simulink model "wheelSuspension"  (R2025a)
settings: Solver=VariableStepAuto  StartTime=0.0  StopTime=10  RelTol=1e-3
undefined symbols (not defined in the file): cs, ks, mass_payload, mass_robot, robot_height
settings Model: DataDictionary=Constants.sldd  Creator=yaremadzulynsky  LastModifiedBy=yaremadzulynsky

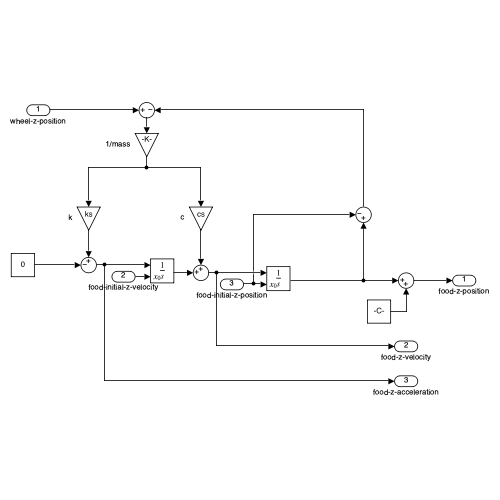
[thumbnail: Simulink's stored preview of the top-level diagram]
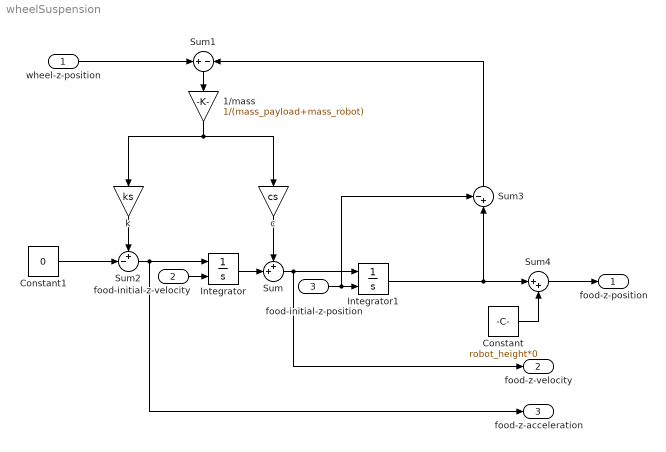
== system wheelSuspension ==
  wheel-z-position : Inport
  food-initial-z-velocity : Inport  Port=2
  food-initial-z-position : Inport  Port=3
  1/mass : Gain  Gain=1/(mass_payload+mass_robot)
  Constant : Constant  Value=robot_height*0
  Constant1 : Constant  Value=0
  Integrator : Integrator  InitialConditionSource=external
  Integrator1 : Integrator  InitialConditionSource=external
  Sum : Sum  Inputs=++|
  Sum1 : Sum  Inputs=+-
  Sum2 : Sum  Inputs=+-|
  Sum3 : Sum  Inputs=-+|
  Sum4 : Sum  Inputs=|++
  c : Gain  Gain=cs
  k : Gain  Gain=ks
  food-z-position : Outport
  food-z-velocity : Outport  Port=2
  food-z-acceleration : Outport  Port=3
  wires:
  Integrator/1 -> Sum/2
  Sum2/1 -> food-z-acceleration/1, Integrator/1
  wheel-z-position/1 -> Sum1/1
  Integrator1/1 -> Sum4/1, Sum3/2
  Sum1/1 -> 1/mass/1
  Sum/1 -> food-z-velocity/1, Integrator1/1
  food-initial-z-velocity/1 -> Integrator/2
  c/1 -> Sum/1
  k/1 -> Sum2/1
  food-initial-z-position/1 -> Sum3/1, Integrator1/2
  1/mass/1 -> k/1, c/1
  Sum3/1 -> Sum1/2
  Sum4/1 -> food-z-position/1
  Constant/1 -> Sum4/2
  Constant1/1 -> Sum2/2
